simulink model "BPF_Activity2"  (R2022a)
settings: Solver=VariableStepAuto  StartTime=0.0  StopTime=10.0  RelTol=1e-3
undefined symbols (not defined in the file or in its folder): fdesignblkfcn, gcbh
libraries: dsparch4 x2, dspsrcs4 x1
settings Model: Creator=chadw  LastModifiedBy=chadw

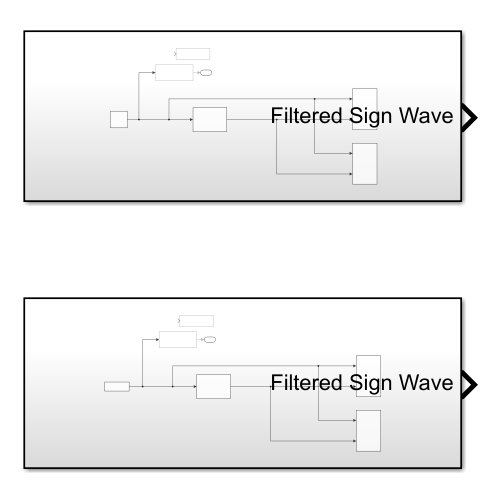
[thumbnail: Simulink's stored preview of the top-level diagram]
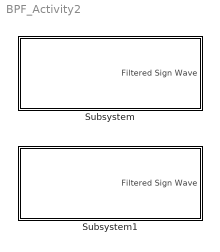
== system BPF_Activity2 ==
  Subsystem : Subsystem
  Subsystem1 : Subsystem

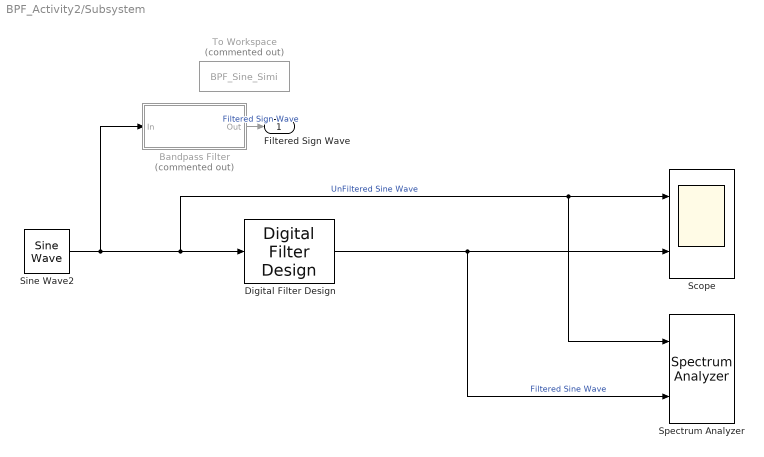
== system BPF_Activity2/Subsystem ==
  Bandpass Filter : Subsystem  Commented=on  DialogController=fdesignblkfcn  InitFcn=fdesignblkfcn(gcbh, {'InitFcn'});  mask(Bandpass Filter){}
      mask help: Design a bandpass filter
      settings: CopyFcn=fdesignblkfcn(gcbh, {'CopyFcn'});
      mask Help: helpview(mapfilelocation('dsp'), 'dspbandpassfilter');
      mask Display: disp('Bandpass');
  Digital Filter Design : dsparch4/Digital Filter Design  mwdsp_browser_bugfix_var=off
  Scope : Scope  NumInputPorts=2
  Sine Wave2 : dspsrcs4/Sine Wave  Amplitude=1  Frequency=100  Phase=0  SampleMode=Discrete  OutComplex=Real  CompMethod=Trigonometric fcn  TableSize=Speed  SampleTime=1/1000  SamplesPerFrame=1  ResetState=Restart at time zero  OutputFrames=off  dataType=double  wordLen=16  udDataType=sfix(16)  fracBitsMode=Best precision  numFracBits=15  OutDataTypeStr=double  LastOutDataTypeStr=double
  Spectrum Analyzer : SpectrumAnalyzer  NumInputPorts=2
  To Workspace : ToWorkspace  Commented=on  VariableName=BPF_Sine_Simi  SaveFormat=Timeseries  SampleTime=-1
  Filtered Sign Wave : Outport
  wires:
  Digital Filter Design/1 -> Spectrum Analyzer/2, Scope/2  "Filtered Sine Wave"
  Sine Wave2/1 -> Bandpass Filter/1(In), Spectrum Analyzer/1, Scope/1, Digital Filter Design/1  "UnFiltered Sine Wave"
  Bandpass Filter/1(Out) -> Filtered Sign Wave/1  "Filtered Sign Wave"

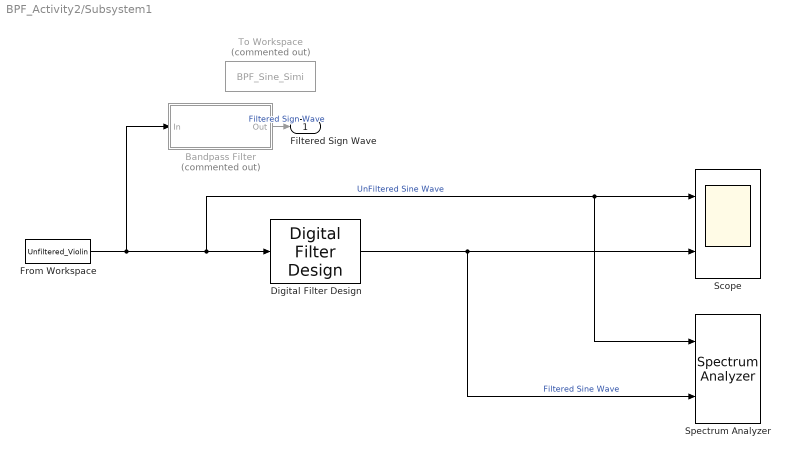
== system BPF_Activity2/Subsystem1 ==
  Bandpass Filter : Subsystem  Commented=on  DialogController=fdesignblkfcn  InitFcn=fdesignblkfcn(gcbh, {'InitFcn'});  mask(Bandpass Filter){}
      mask help: Design a bandpass filter
      settings: CopyFcn=fdesignblkfcn(gcbh, {'CopyFcn'});
      mask Help: helpview(mapfilelocation('dsp'), 'dspbandpassfilter');
      mask Display: disp('Bandpass');
  Digital Filter Design : dsparch4/Digital Filter Design  mwdsp_browser_bugfix_var=off
  From Workspace : FromWorkspace  VariableName=Unfiltered_Violin  SampleTime=-1
  Scope : Scope  NumInputPorts=2
  Spectrum Analyzer : SpectrumAnalyzer  NumInputPorts=2
  To Workspace : ToWorkspace  Commented=on  VariableName=BPF_Sine_Simi  SaveFormat=Timeseries  SampleTime=-1
  Filtered Sign Wave : Outport
  wires:
  Bandpass Filter/1(Out) -> Filtered Sign Wave/1  "Filtered Sign Wave"
  From Workspace/1 -> Digital Filter Design/1, Scope/1, Spectrum Analyzer/1, Bandpass Filter/1(In)  "UnFiltered Sine Wave"
  Digital Filter Design/1 -> Spectrum Analyzer/2, Scope/2  "Filtered Sine Wave"

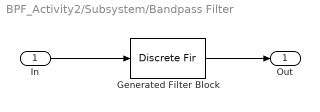
== system BPF_Activity2/Subsystem/Bandpass Filter ==
  In : Inport
  Generated Filter Block : DiscreteFir  Tag=BlockMethodSubSystem  Coefficients=[-0.00089922914877444424 0.00164145187479435928 0.00313520718422255745 -0.00407075508288146874 -0.00637318522279040241 0.00748742868060905172 0.00983543195662957281 -0.0101893165134462078 -0.011302794465874122 0.0096929185841818314 0.00794286539874642684 -0.00313682478812214987 0.00282998788779430157 -0.0115086742430014887 -0.0220801362194615741 0.0342453254245076721 0.0483566616489054524 -0.0623553691698842255 -0.0775034781625938557 0.0906877681531256252 0.103531711058441514 -0.112978600842298299 -0.120358660249784491 0.123793608015391313 0.123793608015391313 -0.120358660249784491 -0.112978600842298299 0.103531711058441514 0.0906877681531256252 -0.0775034781625938557 -0.0623553691698842255 0.0483566616489054524 0.0342453254245076721 -0.0220801362194615741 -0.0115086742430014887 0.00282998788779430157 -0.00313682478812214987 0.00794286539874642684 0.0096929185841818314 -0.011302794465874122 -0.0101893165134462078 0.00983543195662957281 0.00748742868060905172 -0.00637318522279040241 -0.00407075508288146874 0.00313520718422255745 0.00164145187479435928 -0.00089922914877444424]  InputProcessing=Columns as channels (frame based)
  Out : Outport  VectorParamsAs1DForOutWhenUnconnected=off
  wires:
  In/1 -> Generated Filter Block/1
  Generated Filter Block/1 -> Out/1

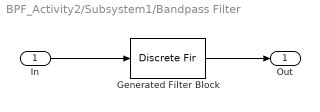
== system BPF_Activity2/Subsystem1/Bandpass Filter ==
  In : Inport
  Generated Filter Block : DiscreteFir  Tag=BlockMethodSubSystem  Coefficients=[-0.00089922914877444424 0.00164145187479435928 0.00313520718422255745 -0.00407075508288146874 -0.00637318522279040241 0.00748742868060905172 0.00983543195662957281 -0.0101893165134462078 -0.011302794465874122 0.0096929185841818314 0.00794286539874642684 -0.00313682478812214987 0.00282998788779430157 -0.0115086742430014887 -0.0220801362194615741 0.0342453254245076721 0.0483566616489054524 -0.0623553691698842255 -0.0775034781625938557 0.0906877681531256252 0.103531711058441514 -0.112978600842298299 -0.120358660249784491 0.123793608015391313 0.123793608015391313 -0.120358660249784491 -0.112978600842298299 0.103531711058441514 0.0906877681531256252 -0.0775034781625938557 -0.0623553691698842255 0.0483566616489054524 0.0342453254245076721 -0.0220801362194615741 -0.0115086742430014887 0.00282998788779430157 -0.00313682478812214987 0.00794286539874642684 0.0096929185841818314 -0.011302794465874122 -0.0101893165134462078 0.00983543195662957281 0.00748742868060905172 -0.00637318522279040241 -0.00407075508288146874 0.00313520718422255745 0.00164145187479435928 -0.00089922914877444424]  InputProcessing=Columns as channels (frame based)
  Out : Outport  VectorParamsAs1DForOutWhenUnconnected=off
  wires:
  Generated Filter Block/1 -> Out/1
  In/1 -> Generated Filter Block/1
